simulink model "Motor_simulink"  (R2024b)
settings: Solver=VariableStepAuto  StartTime=0.0  StopTime=10.0  RelTol=1e-3
InitFcn:
  | R=2;
  | L=23e-9;
  | Ke=0.01;
  | Kt=0.01;
  | b=0.0012;
  | J=0.001;

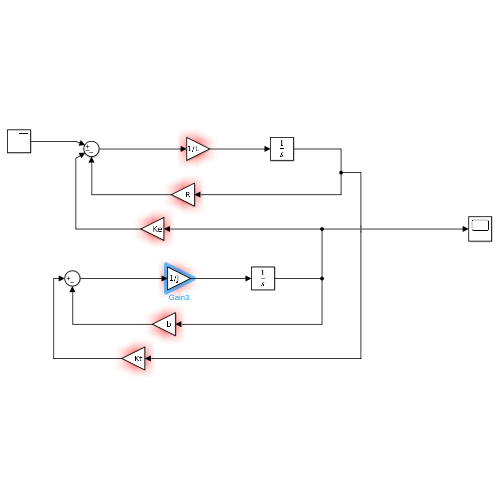
[thumbnail: Simulink's stored preview of the top-level diagram]
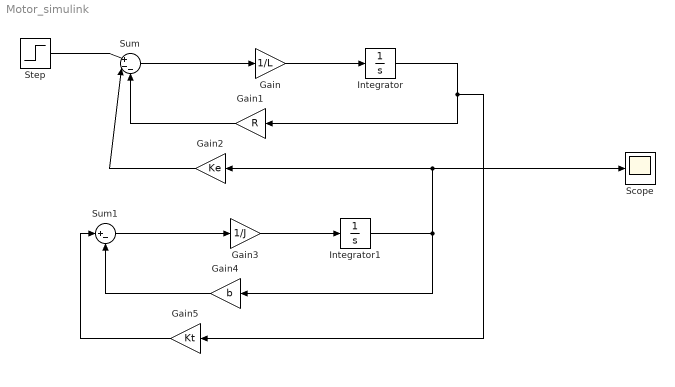
== system Motor_simulink ==
  Gain : Gain  Gain=1/L
  Gain1 : Gain  Gain=R
  Gain2 : Gain  Gain=Ke
  Gain3 : Gain  Gain=1/J
  Gain4 : Gain  Gain=b
  Gain5 : Gain  Gain=Kt
  Integrator : Integrator
  Integrator1 : Integrator
  Scope : Scope
  Step : Step  Time=0  After=5  SampleTime=0
  Sum : Sum  Inputs=|+--
  Sum1 : Sum  Inputs=|+-
  wires:
  Gain/1 -> Integrator/1
  Step/1 -> Sum/1
  Sum/1 -> Gain/1
  Gain1/1 -> Sum/3
  Gain2/1 -> Sum/2
  Integrator/1 -> Gain1/1, Gain5/1
  Gain3/1 -> Integrator1/1
  Sum1/1 -> Gain3/1
  Integrator1/1 -> Gain2/1, Scope/1, Gain4/1
  Gain5/1 -> Sum1/1
  Gain4/1 -> Sum1/2
